simulink library "Aerodynamics"  (R2024a)
settings: Solver=VariableStepAuto  StartTime=0.0  StopTime=10.0  RelTol=1e-3
undefined symbols (not defined in the file): b, c, CD0, CD_Alpha, CD_Elev, CL0, Cl_Ail, CL_Alpha, CL_AlphaDot, Cl_Beta, CL_Elev, Cl_p, CL_q, Cl_r, Cl_Rud, Cm0, Cm_Alpha, Cm_AlphaDot, Cm_Elev, Cm_q, Cn_Ail, Cn_Beta, Cn_p, Cn_r, Cn_Rud, CY_Ail, CY_Beta, CY_p, CY_r, CY_Rud, S, y_CG, z_CG
settings Model: Creator=mahariansyah  LastModifiedBy=mahariansyah

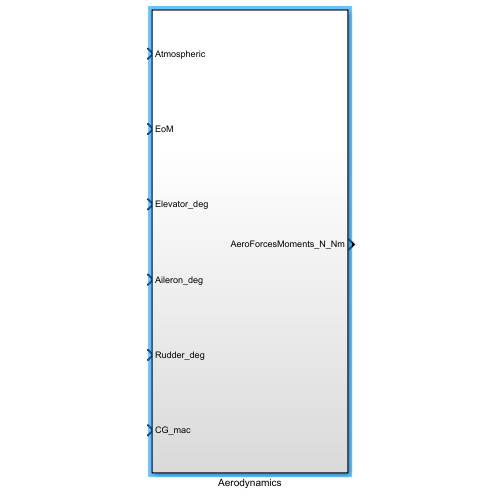
[thumbnail: Simulink's stored preview of the top-level diagram]
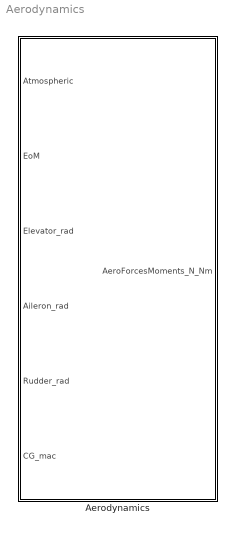
== system Aerodynamics ==
  Aerodynamics : Subsystem

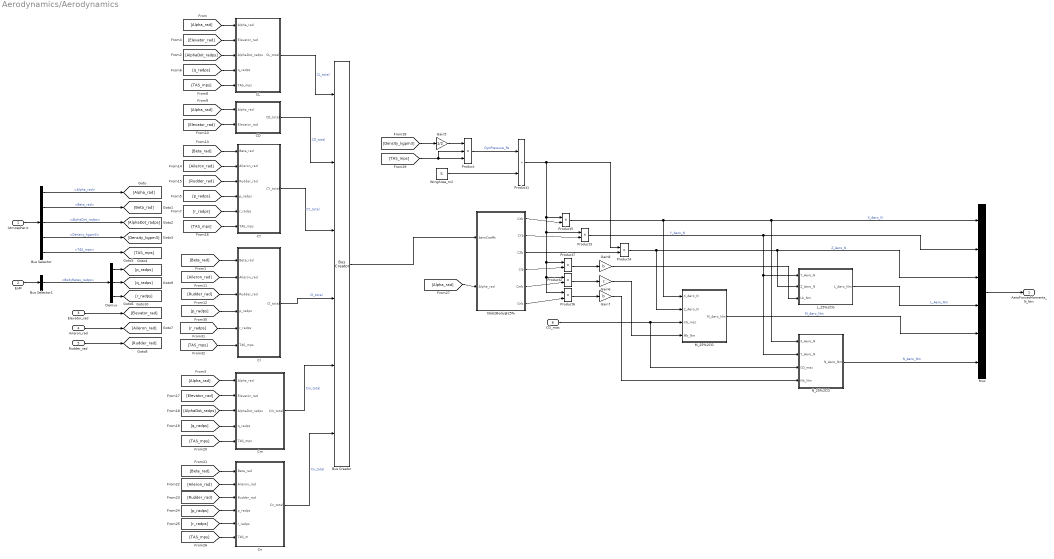
== system Aerodynamics/Aerodynamics ==
  Atmospheric : Inport
  EoM : Inport  Port=2
  Elevator_rad : Inport  Port=3
  Aileron_rad : Inport  Port=4
  Rudder_rad : Inport  Port=5
  CG_mac : Inport  Port=6
  Bus Creator : BusCreator  Inputs=6
  Bus Selector : BusSelector  OutputSignals=Alpha_rad,Beta_rad,AlphaDot_radps,Density_kgpm3,TAS_mps
  Bus Selector1 : BusSelector  OutputSignals=BodyRates_radps
  CD : Subsystem
  CL : Subsystem
  CY : Subsystem
  Cl : Subsystem
  Cm : Subsystem
  Cn : Subsystem
  Demux : Demux  Outputs=3
  Gain5 : Gain  Gain=1/2
  Gain6 : Gain  Gain=c
  Gain7 : Gain  Gain=b
  Gain8 : Gain  Gain=b
  L_25%2CG : Subsystem
  M_25%2CG : Subsystem
  Mux : Mux  Inputs=6
  N_25%2CG : Subsystem
  Product : Product  Inputs=3
  Product{1..7} (7 alike) : Product
  Stab2Body@25% : Subsystem
  WingArea_m2 : Constant  Value=S
  AeroForcesMoments_N_Nm : Outport
  wires:
  Bus Selector/1 -> [Alpha_rad]  "<Alpha_rad>"
  Bus Selector1/1 -> Demux/1  "<BodyRates_radps>"
  EoM/1 -> Bus Selector1/1
  Atmospheric/1 -> Bus Selector/1
  [q_radps] -> CL/4(q_radps)
  Rudder_rad/1 -> [Rudder_rad]
  [Aileron_rad] -> Cl/2(Aileron_rad)
  [Elevator_rad] -> Cm/2(Elevator_rad)
  [TAS_mps] -> CL/5(TAS_mps)
  CL/1(CL_total) -> Bus Creator/1  "CL_total"
  [p_radps] -> CY/4(p_radps)
  Cn/1(Cn_total) -> Bus Creator/6  "Cn_total"
  [Alpha_rad] -> CL/1(Alpha_rad)
  Stab2Body@25%/2(CYb) -> Product3/2
  [Elevator_rad] -> CD/2(Elevator_rad)
  Stab2Body@25%/6(Cnb) -> Product6/2
  Bus Selector/5 -> [TAS_mps]  "<TAS_mps>"
  [Aileron_rad] -> Cn/2(Aileron_rad)
  [Density_kgpm3] -> Gain5/1
  Aileron_rad/1 -> [Aileron_rad]
  [Alpha_rad] -> Stab2Body@25%/2(Alpha_rad)
  [TAS_mps] -> Product/2, Product/3
  [AlphaDot_radps] -> CL/3(AlphaDot_radps)
  [Beta_rad] -> CY/1(Beta_rad)
  [AlphaDot_radps] -> Cm/3(AlphaDot_radps)
  Bus Selector/2 -> [Beta_rad]  "<Beta_rad>"
  [q_radps] -> Cm/4(q_radps)
  [Alpha_rad] -> Cm/1(Alpha_rad)
  Stab2Body@25%/5(Cmb) -> Product2/2
  [Rudder_rad] -> Cn/3(Rudder_rad)
  [p_radps] -> Cn/4(p_radps)
  Product5/1 -> Mux/1, N_25%2CG/1(X_Aero_N), M_25%2CG/1(X_Aero_N)  "X_Aero_N"
  [Beta_rad] -> Cl/1(Beta_rad)
  [Rudder_rad] -> CY/3(Rudder_rad)
  Stab2Body@25%/3(CZb) -> Product4/2
  Bus Selector/3 -> [AlphaDot_radps]  "<AlphaDot_radps>"
  WingArea_m2/1 -> Product1/2
  [Alpha_rad] -> CD/1(Alpha_rad)
  [Elevator_rad] -> CL/2(Elevator_rad)
  CD/1(CD_total) -> Bus Creator/2  "CD_total"
  [TAS_mps] -> CY/6(TAS_mps)
  [r_radps] -> CY/5(r_radps)
  Product/1 -> Product1/1  "DynPressure_Pa"
  Product3/1 -> N_25%2CG/2(Y_Aero_N), L_25%2CG/1(Y_Aero_N), Mux/2  "Y_Aero_N"
  Product2/1 -> Gain6/1
  [TAS_mps] -> Cn/6(TAS_m)
  [Rudder_rad] -> Cl/3(Rudder_rad)
  Demux/3 -> [r_radps]
  Demux/1 -> [p_radps]
  [r_radps] -> Cn/5(r_radps)
  Product7/1 -> Gain8/1
  Product1/1 -> Product5/1, Product3/1, Product6/1, Product2/1, Product7/1, Product4/1
  Stab2Body@25%/4(Clb) -> Product7/2
  Cm/1(Cm_total) -> Bus Creator/5  "Cm_total"
  CY/1(CY_total) -> Bus Creator/3  "CY_total"
  Gain7/1 -> N_25%2CG/4(Nb_Nm)
  Bus Selector/4 -> [Density_kgpm3]  "<Density_kgpm3>"
  Product6/1 -> Gain7/1
  Stab2Body@25%/1(CXb) -> Product5/2
  [Aileron_rad] -> CY/2(Aileron_rad)
  [TAS_mps] -> Cm/5(TAS_mps)
  CG_mac/1 -> N_25%2CG/3(CG_mac), M_25%2CG/3(CG_mac)
  Gain8/1 -> L_25%2CG/3(Lb_Nm)
  Gain6/1 -> M_25%2CG/4(Mb_Nm)
  Product4/1 -> Mux/3, L_25%2CG/2(Z_Aero_N), M_25%2CG/2(Z_Aero_N)  "Z_Aero_N"
  Bus Creator/1 -> Stab2Body@25%/1(AeroCoeffs)
  L_25%2CG/1(L_Aero_Nm) -> Mux/4  "L_Aero_Nm"
  Demux/2 -> [q_radps]
  Cl/1(Cl_total) -> Bus Creator/4  "Cl_total"
  [Beta_rad] -> Cn/1(Beta_rad)
  M_25%2CG/1(M_Aero_Nm) -> Mux/5  "M_Aero_Nm"
  Mux/1 -> AeroForcesMoments_N_Nm/1
  N_25%2CG/1(N_Aero_Nm) -> Mux/6  "N_Aero_Nm"
  Elevator_rad/1 -> [Elevator_rad]
  Gain5/1 -> Product/1
  [TAS_mps] -> Cl/6(TAS_mps)
  [r_radps] -> Cl/5(r_radps)
  [p_radps] -> Cl/4(p_radps)

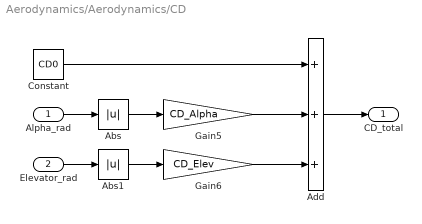
== system Aerodynamics/Aerodynamics/CD ==
  Alpha_rad : Inport
  Elevator_rad : Inport  Port=2
  Abs : Abs  SaturateOnIntegerOverflow=off
  Abs1 : Abs  SaturateOnIntegerOverflow=off
  Add : Sum  Inputs=+++
  Constant : Constant  Value=CD0
  Gain5 : Gain  Gain=CD_Alpha
  Gain6 : Gain  Gain=CD_Elev
  CD_total : Outport
  wires:
  Constant/1 -> Add/1
  Elevator_rad/1 -> Abs1/1
  Alpha_rad/1 -> Abs/1
  Gain5/1 -> Add/2
  Gain6/1 -> Add/3
  Add/1 -> CD_total/1
  Abs/1 -> Gain5/1
  Abs1/1 -> Gain6/1

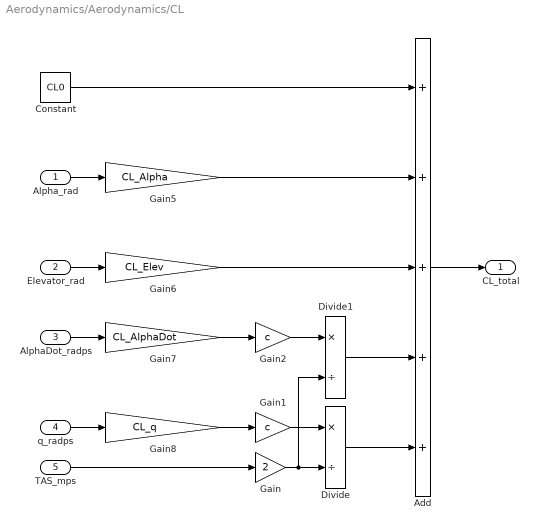
== system Aerodynamics/Aerodynamics/CL ==
  Alpha_rad : Inport
  Elevator_rad : Inport  Port=2
  AlphaDot_radps : Inport  Port=3
  q_radps : Inport  Port=4
  TAS_mps : Inport  Port=5
  Add : Sum  Inputs=+++++
  Constant : Constant  Value=CL0
  Divide : Product  Inputs=*/
  Divide1 : Product  Inputs=*/
  Gain : Gain  Gain=2
  Gain1 : Gain  Gain=c
  Gain2 : Gain  Gain=c
  Gain5 : Gain  Gain=CL_Alpha
  Gain6 : Gain  Gain=CL_Elev
  Gain7 : Gain  Gain=CL_AlphaDot
  Gain8 : Gain  Gain=CL_q
  CL_total : Outport
  wires:
  AlphaDot_radps/1 -> Gain7/1
  q_radps/1 -> Gain8/1
  Alpha_rad/1 -> Gain5/1
  Elevator_rad/1 -> Gain6/1
  Gain5/1 -> Add/2
  Gain6/1 -> Add/3
  Constant/1 -> Add/1
  Add/1 -> CL_total/1
  TAS_mps/1 -> Gain/1
  Gain/1 -> Divide1/2, Divide/2
  Gain8/1 -> Gain1/1
  Gain1/1 -> Divide/1
  Divide/1 -> Add/5
  Gain2/1 -> Divide1/1
  Gain7/1 -> Gain2/1
  Divide1/1 -> Add/4

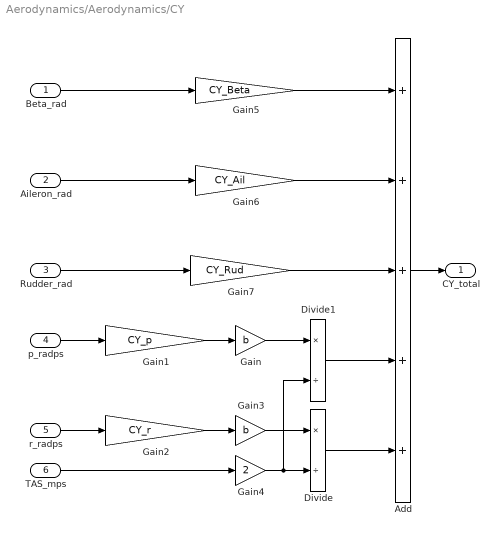
== system Aerodynamics/Aerodynamics/CY ==
  Beta_rad : Inport
  Aileron_rad : Inport  Port=2
  Rudder_rad : Inport  Port=3
  p_radps : Inport  Port=4
  r_radps : Inport  Port=5
  TAS_mps : Inport  Port=6
  Add : Sum  Inputs=+++++
  Divide : Product  Inputs=*/
  Divide1 : Product  Inputs=*/
  Gain : Gain  Gain=b
  Gain1 : Gain  Gain=CY_p
  Gain2 : Gain  Gain=CY_r
  Gain3 : Gain  Gain=b
  Gain4 : Gain  Gain=2
  Gain5 : Gain  Gain=CY_Beta
  Gain6 : Gain  Gain=CY_Ail
  Gain7 : Gain  Gain=CY_Rud
  CY_total : Outport
  wires:
  Rudder_rad/1 -> Gain7/1
  Gain7/1 -> Add/3
  Beta_rad/1 -> Gain5/1
  Gain6/1 -> Add/2
  Aileron_rad/1 -> Gain6/1
  Gain5/1 -> Add/1
  Add/1 -> CY_total/1
  p_radps/1 -> Gain1/1
  Gain1/1 -> Gain/1
  r_radps/1 -> Gain2/1
  Gain2/1 -> Gain3/1
  TAS_mps/1 -> Gain4/1
  Gain3/1 -> Divide/1
  Gain4/1 -> Divide1/2, Divide/2
  Divide/1 -> Add/5
  Divide1/1 -> Add/4
  Gain/1 -> Divide1/1

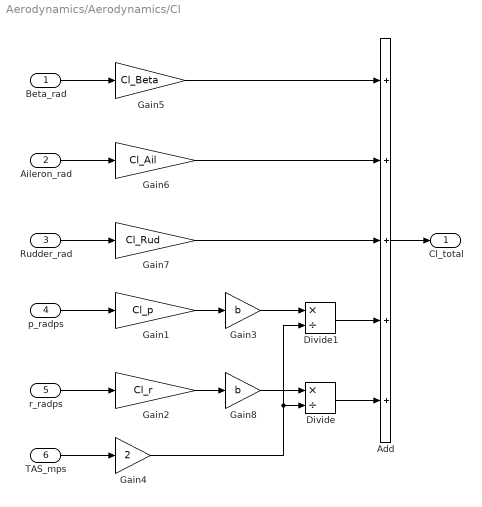
== system Aerodynamics/Aerodynamics/Cl ==
  Beta_rad : Inport
  Aileron_rad : Inport  Port=2
  Rudder_rad : Inport  Port=3
  p_radps : Inport  Port=4
  r_radps : Inport  Port=5
  TAS_mps : Inport  Port=6
  Add : Sum  Inputs=+++++
  Divide : Product  Inputs=*/
  Divide1 : Product  Inputs=*/
  Gain1 : Gain  Gain=Cl_p
  Gain2 : Gain  Gain=Cl_r
  Gain3 : Gain  Gain=b
  Gain4 : Gain  Gain=2
  Gain5 : Gain  Gain=Cl_Beta
  Gain6 : Gain  Gain=Cl_Ail
  Gain7 : Gain  Gain=Cl_Rud
  Gain8 : Gain  Gain=b
  Cl_total : Outport
  wires:
  Gain6/1 -> Add/2
  Gain5/1 -> Add/1
  Aileron_rad/1 -> Gain6/1
  Beta_rad/1 -> Gain5/1
  Rudder_rad/1 -> Gain7/1
  Gain7/1 -> Add/3
  Add/1 -> Cl_total/1
  p_radps/1 -> Gain1/1
  Gain1/1 -> Gain3/1
  TAS_mps/1 -> Gain4/1
  Gain2/1 -> Gain8/1
  r_radps/1 -> Gain2/1
  Divide/1 -> Add/5
  Gain8/1 -> Divide/1
  Gain4/1 -> Divide1/2, Divide/2
  Divide1/1 -> Add/4
  Gain3/1 -> Divide1/1

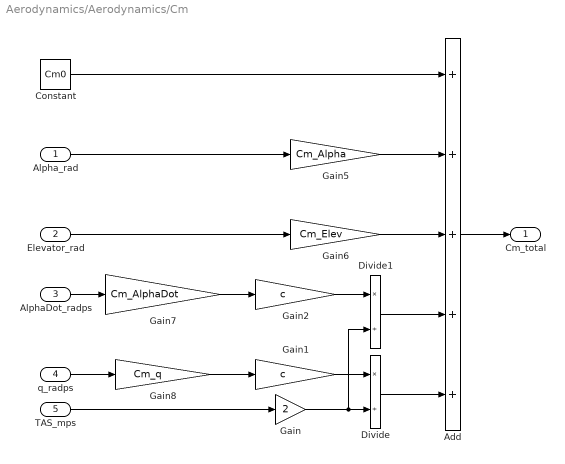
== system Aerodynamics/Aerodynamics/Cm ==
  Alpha_rad : Inport
  Elevator_rad : Inport  Port=2
  AlphaDot_radps : Inport  Port=3
  q_radps : Inport  Port=4
  TAS_mps : Inport  Port=5
  Add : Sum  Inputs=+++++
  Constant : Constant  Value=Cm0
  Divide : Product  Inputs=*/
  Divide1 : Product  Inputs=*/
  Gain : Gain  Gain=2
  Gain1 : Gain  Gain=c
  Gain2 : Gain  Gain=c
  Gain5 : Gain  Gain=Cm_Alpha
  Gain6 : Gain  Gain=Cm_Elev
  Gain7 : Gain  Gain=Cm_AlphaDot
  Gain8 : Gain  Gain=Cm_q
  Cm_total : Outport
  wires:
  Gain8/1 -> Gain1/1
  Gain6/1 -> Add/3
  Elevator_rad/1 -> Gain6/1
  AlphaDot_radps/1 -> Gain7/1
  q_radps/1 -> Gain8/1
  Gain5/1 -> Add/2
  Alpha_rad/1 -> Gain5/1
  Constant/1 -> Add/1
  TAS_mps/1 -> Gain/1
  Gain/1 -> Divide1/2, Divide/2
  Gain1/1 -> Divide/1
  Divide/1 -> Add/5
  Divide1/1 -> Add/4
  Gain2/1 -> Divide1/1
  Gain7/1 -> Gain2/1
  Add/1 -> Cm_total/1

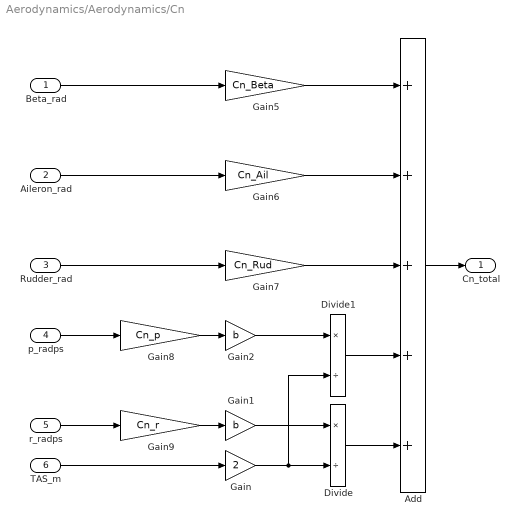
== system Aerodynamics/Aerodynamics/Cn ==
  Beta_rad : Inport
  Aileron_rad : Inport  Port=2
  Rudder_rad : Inport  Port=3
  p_radps : Inport  Port=4
  r_radps : Inport  Port=5
  TAS_m : Inport  Port=6
  Add : Sum  Inputs=+++++
  Divide : Product  Inputs=*/
  Divide1 : Product  Inputs=*/
  Gain : Gain  Gain=2
  Gain1 : Gain  Gain=b
  Gain2 : Gain  Gain=b
  Gain5 : Gain  Gain=Cn_Beta
  Gain6 : Gain  Gain=Cn_Ail
  Gain7 : Gain  Gain=Cn_Rud
  Gain8 : Gain  Gain=Cn_p
  Gain9 : Gain  Gain=Cn_r
  Cn_total : Outport
  wires:
  Rudder_rad/1 -> Gain7/1
  r_radps/1 -> Gain9/1
  Gain5/1 -> Add/1
  p_radps/1 -> Gain8/1
  Gain7/1 -> Add/3
  Beta_rad/1 -> Gain5/1
  Aileron_rad/1 -> Gain6/1
  Gain6/1 -> Add/2
  TAS_m/1 -> Gain/1
  Gain/1 -> Divide1/2, Divide/2
  Gain9/1 -> Gain1/1
  Gain1/1 -> Divide/1
  Divide/1 -> Add/5
  Divide1/1 -> Add/4
  Gain2/1 -> Divide1/1
  Gain8/1 -> Gain2/1
  Add/1 -> Cn_total/1

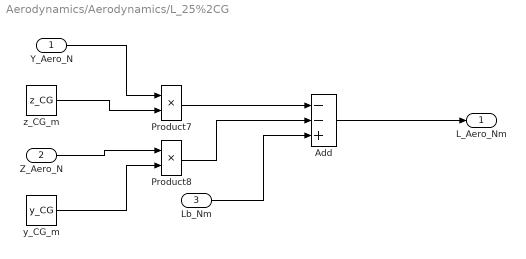
== system Aerodynamics/Aerodynamics/L_25%2CG ==
  Y_Aero_N : Inport
  Z_Aero_N : Inport  Port=2
  Lb_Nm : Inport  Port=3
  Add : Sum  Inputs=--+
  Product7 : Product
  Product8 : Product
  y_CG_m : Constant  Value=y_CG
  z_CG_m : Constant  Value=z_CG
  L_Aero_Nm : Outport
  wires:
  Product7/1 -> Add/1
  Lb_Nm/1 -> Add/3
  Z_Aero_N/1 -> Product8/1
  z_CG_m/1 -> Product7/2
  Product8/1 -> Add/2
  Y_Aero_N/1 -> Product7/1
  y_CG_m/1 -> Product8/2
  Add/1 -> L_Aero_Nm/1

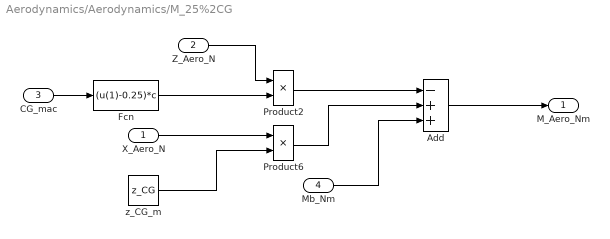
== system Aerodynamics/Aerodynamics/M_25%2CG ==
  X_Aero_N : Inport
  Z_Aero_N : Inport  Port=2
  CG_mac : Inport  Port=3
  Mb_Nm : Inport  Port=4
  Add : Sum  Inputs=-++
  Fcn : Fcn  Expr=(u(1)-0.25)*c
  Product2 : Product
  Product6 : Product
  z_CG_m : Constant  Value=z_CG
  M_Aero_Nm : Outport
  wires:
  X_Aero_N/1 -> Product6/1
  z_CG_m/1 -> Product6/2
  Add/1 -> M_Aero_Nm/1
  CG_mac/1 -> Fcn/1
  Z_Aero_N/1 -> Product2/1
  Fcn/1 -> Product2/2
  Product2/1 -> Add/1
  Product6/1 -> Add/2
  Mb_Nm/1 -> Add/3

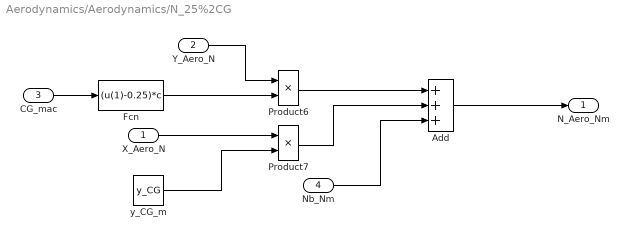
== system Aerodynamics/Aerodynamics/N_25%2CG ==
  X_Aero_N : Inport
  Y_Aero_N : Inport  Port=2
  CG_mac : Inport  Port=3
  Nb_Nm : Inport  Port=4
  Add : Sum  Inputs=+++
  Fcn : Fcn  Expr=(u(1)-0.25)*c
  Product6 : Product
  Product7 : Product
  y_CG_m : Constant  Value=y_CG
  N_Aero_Nm : Outport
  wires:
  y_CG_m/1 -> Product7/2
  CG_mac/1 -> Fcn/1
  Add/1 -> N_Aero_Nm/1
  Product6/1 -> Add/1
  X_Aero_N/1 -> Product7/1
  Y_Aero_N/1 -> Product6/1
  Nb_Nm/1 -> Add/3
  Product7/1 -> Add/2
  Fcn/1 -> Product6/2

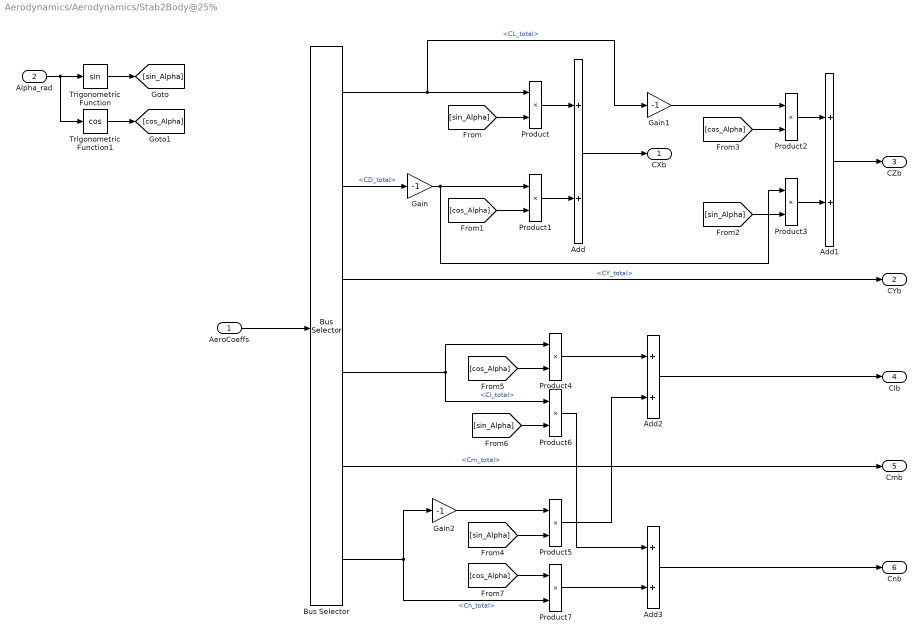
== system Aerodynamics/Aerodynamics/Stab2Body@25% ==
  AeroCoeffs : Inport
  Alpha_rad : Inport  Port=2
  Add{,1..3} (4 alike) : Sum
  Bus Selector : BusSelector  OutputSignals=CL_total,CD_total,CY_total,Cl_total,Cm_total,Cn_total
  Gain : Gain  Gain=-1
  Gain1 : Gain  Gain=-1
  Gain2 : Gain  Gain=-1
  Product{,1..7} (8 alike) : Product
  Trigonometric Function : Trigonometry
  Trigonometric Function1 : Trigonometry  Operator=cos
  CXb : Outport
  CYb : Outport  Port=2
  CZb : Outport  Port=3
  Clb : Outport  Port=4
  Cmb : Outport  Port=5
  Cnb : Outport  Port=6
  wires:
  AeroCoeffs/1 -> Bus Selector/1
  Alpha_rad/1 -> Trigonometric Function1/1, Trigonometric Function/1
  Trigonometric Function/1 -> [sin_Alpha]
  Trigonometric Function1/1 -> [cos_Alpha]
  Bus Selector/1 -> Gain1/1, Product/1  "<CL_total>"
  Bus Selector/2 -> Gain/1  "<CD_total>"
  Bus Selector/3 -> CYb/1  "<CY_total>"
  [sin_Alpha] -> Product/2
  Gain/1 -> Product3/1, Product1/1
  [cos_Alpha] -> Product1/2
  Product/1 -> Add/1
  Product1/1 -> Add/2
  Add/1 -> CXb/1
  Product3/1 -> Add1/2
  Product2/1 -> Add1/1
  Gain1/1 -> Product2/1
  [cos_Alpha] -> Product2/2
  [sin_Alpha] -> Product3/2
  Add1/1 -> CZb/1
  Bus Selector/4 -> Product6/1, Product4/1  "<Cl_total>"
  Bus Selector/5 -> Cmb/1  "<Cm_total>"
  Bus Selector/6 -> Product7/2, Gain2/1  "<Cn_total>"
  Product7/1 -> Add3/2
  Product6/1 -> Add3/1
  Add3/1 -> Cnb/1
  [cos_Alpha] -> Product7/1
  Add2/1 -> Clb/1
  Product5/1 -> Add2/2
  [sin_Alpha] -> Product6/2
  [cos_Alpha] -> Product4/2
  Product4/1 -> Add2/1
  Gain2/1 -> Product5/1
  [sin_Alpha] -> Product5/2
